simulink subsystem "Final_Project_PreRealSurface_20260605_142446"  (R2024a)
settings: Solver=VariableStepAuto  StartTime=0.0  StopTime=10.0  RelTol=1e-3
values from neighbouring files (symbols this model uses):
  D = hypot(Ep(:,1)-Tp(:,1)',Ep(:,2)-Tp(:,2)')    [pp_compare_stage.m]    (also in pp_diag_path.m; pp_t09_clear.m = hypot(Ep(:,1)-Tperim(:,1)', Ep(:,2)-Tperim(:,2)'); pp_tune2.m)
undefined symbols (not defined in the file or in its folder): waypoint_const
libraries: CarMaker4SL x83, simulink x2
(part 1 of 5)
settings Model: Creator=junho.lee  LastModifiedBy=hajin

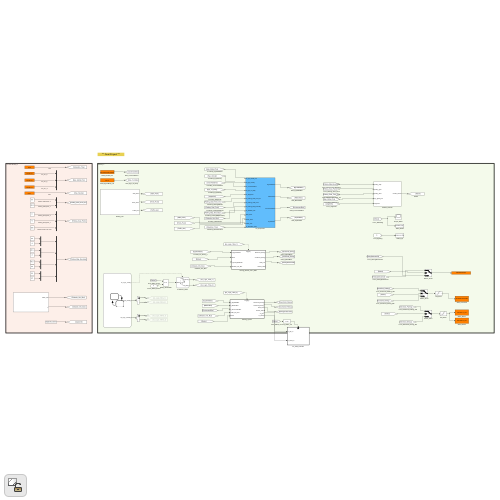
[thumbnail: Simulink's stored preview of the top-level diagram]
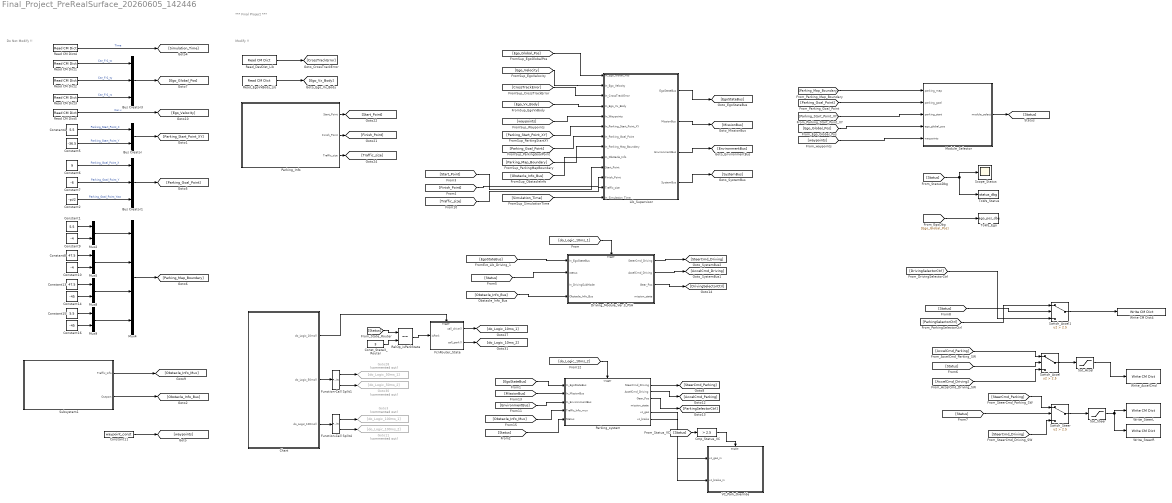
== system Final_Project_PreRealSurface_20260605_142446 ==
  note: Do Not Modify !!
  note: *** Final Project ***
  note: Modify !!
  Bus Creator : BusCreator  Inputs=2
  Bus Creator1 : BusCreator  Inputs=3
  Bus Creator3 : BusCreator  Inputs=3
  Chart : Stateflow chart  TreatAsAtomicUnit=on
  Cmp_Status_VC : simulink/Logic and Bit Operations/Compare To Constant  relop=>  const=2.5  OutDataTypeStr=boolean
  Const_State3_Router : Constant  Value=3
  Constant1 : Constant  Value=5.5
  Constant10 : Constant  Value=-4
  Constant11 : Constant  Value=waypoint_const
  Constant13 : Constant  Value=47.5
  Constant14 : Constant  Value=-45
  Constant15 : Constant  Value=5.5
  Constant16 : Constant  Value=-45
  Constant2 : Constant  Value=-pi/2
  Constant4 : Constant  Value=5.5
  Constant5 : Constant  Value=-36.5
  Constant6 : Constant  Value=9
  Constant7 : Constant  Value=-6
  Constant8 : Constant  Value=47.5
  Constant9 : Constant  Value=-4
  Driving_Module_Ver.3_PSH : Subsystem
  FcnRouter_State : Stateflow chart  TreatAsAtomicUnit=on
  Function-Call Split1 : FunctionCallSplit  IconShape=distinctive  NumOutputPorts=2  OutputPortLayout=default
  Function-Call Split4 : FunctionCallSplit  IconShape=distinctive  NumOutputPorts=2  OutputPortLayout=default
  Goto11 : Goto  Commented=on  GotoTag=do_Logic_100ms_2
  Goto28 : Goto  Commented=on  GotoTag=do_Logic_50ms_1
  Goto3 : Goto  Commented=on  GotoTag=do_Logic_100ms_1
  Goto30 : Goto  Commented=on  GotoTag=do_Logic_50ms_2
  Lib_Supervisor : Subsystem
  Module_Selector : Subsystem
  Mux{2,5,8..9} (4 alike) : Mux  Inputs=2
  Mux4 : Mux
  Parking_Info : Subsystem
  Parking_system : Subsystem
  Read CM Dict1 : CarMaker4SL/Read CM Dict  xname=Car.Fr1.tx  xsync=off  xstime=Inherited
  Read CM Dict2 : CarMaker4SL/Read CM Dict  xname=Car.Fr1.ty  xsync=off  xstime=Inherited
  Read CM Dict3 : CarMaker4SL/Read CM Dict  xname=Car.Fr1.rz  xsync=off  xstime=Inherited
  Read CM Dict4 : CarMaker4SL/Read CM Dict  xname=Time  xsync=off  xstime=Inherited
  Read CM Dict5 : CarMaker4SL/Read CM Dict  xname=Car.v  xsync=off  xstime=Inherited
  Read_DevDist_Lib : CarMaker4SL/Read CM Dict  xname=Car.Road.Path.DevDist  xsync=off  xstime=Inherited
  Read_EgoVxBody_Lib : CarMaker4SL/Read CM Dict  xname=Car.vx  xsync=off  xstime=Inherited
  RelOp_isParkState : RelationalOperator  Operator===
  Sat_Accel : Saturate  UpperLimit=3.0  LowerLimit=-5.0
  Sat_Steer : Saturate  UpperLimit=pi/6  LowerLimit=-pi/6
  Scope_Status : Scope
  Subsystem1 : Subsystem
  Switch_Accel : Switch  Criteria=u2 > Threshold  Threshold=2.5
  Switch_Accel1 : Switch  Criteria=u2 > Threshold  Threshold=2.5
  Switch_Steer : Switch  Criteria=u2 > Threshold  Threshold=2.5
  ToWs_Ego : ToWorkspace  VariableName=ego_pos_dbg  SaveFormat=Timeseries  SampleTime=-1
  ToWs_Status : ToWorkspace  VariableName=status_dbg  SaveFormat=Timeseries  SampleTime=-1
  VC_Park_Override : Subsystem
  Write CM Dict4 : CarMaker4SL/Write CM Dict  xname=DM.SelectorCtrl  xsync=off
  Write_AccelCmd : CarMaker4SL/Write CM Dict  xname=AccelCtrl.DesiredAx  xsync=off
  Write_SteerL : CarMaker4SL/Write CM Dict  xname=Car.CFL.rz_ext  xsync=off
  Write_SteerR : CarMaker4SL/Write CM Dict  xname=Car.CFR.rz_ext  xsync=off
  wires:
  Constant13/1 -> Mux8/1
  Subsystem1/1(Traffic_Info) -> [Obstacle_Info_Mux]
  Read CM Dict1/1 -> Bus Creator3/1  "Car_Fr1_tx"
  Read CM Dict3/1 -> Bus Creator3/3  "Car_Fr1_rz"
  Constant4/1 -> Bus Creator/1  "Parking_Start_Point_X"
  Chart/2(do_Logic_50ms()) -> Function-Call Split1/1
  Function-Call Split1/2 -> Goto30/1
  Read CM Dict4/1 -> [Simulation_Time]  "Time"
  Constant9/1 -> Mux2/2
  Bus Creator1/1 -> [Parking_Goal_Point]
  Mux8/1 -> Mux4/3
  Constant6/1 -> Bus Creator1/1  "Parking_Goal_Point_X"
  Constant1/1 -> Mux2/1
  Constant16/1 -> Mux9/2
  Read CM Dict2/1 -> Bus Creator3/2  "Car_Fr1_ty"
  Function-Call Split1/1 -> Goto28/1
  Constant5/1 -> Bus Creator/2  "Parking_Start_Point_Y"
  Constant7/1 -> Bus Creator1/2  "Parking_Goal_Point_Y"
  Read CM Dict5/1 -> [Ego_Velocity]  "Car.v"
  Constant15/1 -> Mux9/1
  Constant10/1 -> Mux5/2
  Bus Creator3/1 -> [Ego_Global_Pos]
  Constant14/1 -> Mux8/2
  Bus Creator/1 -> [Parking_Start_Point_XY]
  Mux9/1 -> Mux4/4
  Mux2/1 -> Mux4/1
  Mux4/1 -> [Parking_Map_Boundary]
  Constant8/1 -> Mux5/1
  Constant2/1 -> Bus Creator1/3  "Parking_Goal_Point_Yaw"
  Mux5/1 -> Mux4/2
  Chart/3(do_Logic_100ms()) -> Function-Call Split4/1
  Function-Call Split4/1 -> Goto3/1
  Function-Call Split4/2 -> Goto11/1
  Sat_Steer/1 -> Write_SteerR/1, Write_SteerL/1
  Read_DevDist_Lib/1 -> [CrossTrackError]
  Read_EgoVxBody_Lib/1 -> [Ego_Vx_Body]
  [Ego_Global_Pos] -> Lib_Supervisor/1(In_Ego_Global_Pos)
  [Ego_Velocity] -> Lib_Supervisor/2(In_Ego_Velocity)
  [CrossTrackError] -> Lib_Supervisor/3(In_CrossTrackError)
  [Ego_Vx_Body] -> Lib_Supervisor/4(In_Ego_Vx_Body)
  [waypoints] -> Lib_Supervisor/5(In_Waypoints)
  [Parking_Start_Point_XY] -> Lib_Supervisor/6(In_Parking_Start_Point_XY)
  [Parking_Goal_Point] -> Lib_Supervisor/7(In_Parking_Goal_Point)
  [Parking_Map_Boundary] -> Lib_Supervisor/8(In_Parking_Map_Boundary)
  [Simulation_Time] -> Lib_Supervisor/13(In_Simulation_Time)
  Lib_Supervisor/1(EgoStateBus) -> [EgoStateBus]
  Lib_Supervisor/2(MissionBus) -> [MissionBus]
  Lib_Supervisor/3(EnvironmentBus) -> [EnvironmentBus]
  Lib_Supervisor/4(SystemBus) -> [SystemBus]
  [EgoStateBus] -> Driving_Module_Ver.3_PSH/1(In_EgoStateBus)
  [do_Logic_10ms_1] -> Driving_Module_Ver.3_PSH/Trigger
  [SteerCmd_Parking] -> Switch_Steer/1
  [Status] -> Switch_Steer/2
  [SteerCmd_Driving] -> Switch_Steer/3
  Switch_Steer/1 -> Sat_Steer/1
  [AccelCmd_Parking] -> Switch_Accel/1
  [Status] -> Switch_Accel/2
  [AccelCmd_Driving] -> Switch_Accel/3
  Switch_Accel/1 -> Sat_Accel/1
  Switch_Accel1/1 -> Write CM Dict4/1
  Sat_Accel/1 -> Write_AccelCmd/1
  Subsystem1/2(Outport) -> [Obstacle_Info_Bus]
  [Obstacle_Info_Bus] -> Lib_Supervisor/9(In_Obstacle_Info)
  Driving_Module_Ver.3_PSH/1(SteerCmd_Driving) -> [SteerCmd_Driving]
  Driving_Module_Ver.3_PSH/2(AccelCmd_Driving) -> [AccelCmd_Driving]
  [Obstacle_Info_Bus] -> Driving_Module_Ver.3_PSH/4(Obstacle_Info_Bus)
  Driving_Module_Ver.3_PSH/3(Gear_Pos) -> [DrivingSelectorCtrl]
  Parking_Info/1(Start_Point) -> [Start_Point]
  Parking_Info/2(Finish_Point) -> [Finish_Point]
  Parking_Info/3(Traffic_size) -> [Traffic_size]
  [Start_Point] -> Lib_Supervisor/10(Start_Point)
  [Finish_Point] -> Lib_Supervisor/11(Finish_Point)
  [Traffic_size] -> Lib_Supervisor/12(Traffic_size)
  [do_Logic_10ms_2] -> Parking_system/Trigger
  [EgoStateBus] -> Parking_system/1(In_EgoStateBus)
  [EnvironmentBus] -> Parking_system/3(In_EnvironmentBus)
  [MissionBus] -> Parking_system/2(In_MissionBus)
  [Obstacle_Info_Mux] -> Parking_system/4(Traffic_Info_mux)
  [Status] -> Driving_Module_Ver.3_PSH/2(status)
  [Parking_Map_Boundary] -> Module_Selector/1(parking_map)
  [Parking_Goal_Point] -> Module_Selector/2(parking_goal)
  [Parking_Start_Point_XY] -> Module_Selector/3(parking_start)
  [Ego_Global_Pos] -> Module_Selector/4(ego_global_pos)
  [waypoints] -> Module_Selector/5(waypoints)
  Module_Selector/1(module_select) -> [Status]
  [Status] -> Parking_system/5(Status)
  Constant11/1 -> [waypoints]
  [Status] -> Scope_Status/1, ToWs_Status/1
  [Ego_Global_Pos] -> ToWs_Ego/1
  [Status] -> RelOp_isParkState/1
  Const_State3_Router/1 -> RelOp_isParkState/2
  Chart/1(do_Logic_10ms()) -> FcnRouter_State/Trigger
  RelOp_isParkState/1 -> FcnRouter_State/1(isPark)
  FcnRouter_State/1(call_drive()) -> [do_Logic_10ms_1]
  FcnRouter_State/2(call_park()) -> [do_Logic_10ms_2]
  [Status] -> Switch_Accel1/2
  Parking_system/1(SteerCmd_Driving) -> [SteerCmd_Parking]
  Parking_system/2(AccelCmd_Driving) -> [AccelCmd_Parking]
  Parking_system/3(Gear_Pos) -> [ParkingSelectorCtrl]
  [ParkingSelectorCtrl] -> Switch_Accel1/1
  [DrivingSelectorCtrl] -> Switch_Accel1/3
  [Status] -> Cmp_Status_VC/1
  Cmp_Status_VC/1 -> VC_Park_Override/Enable
  Parking_system/5(vc_gas) -> VC_Park_Override/1(vc_gas_in)
  Parking_system/6(vc_brake) -> VC_Park_Override/2(vc_brake_in)

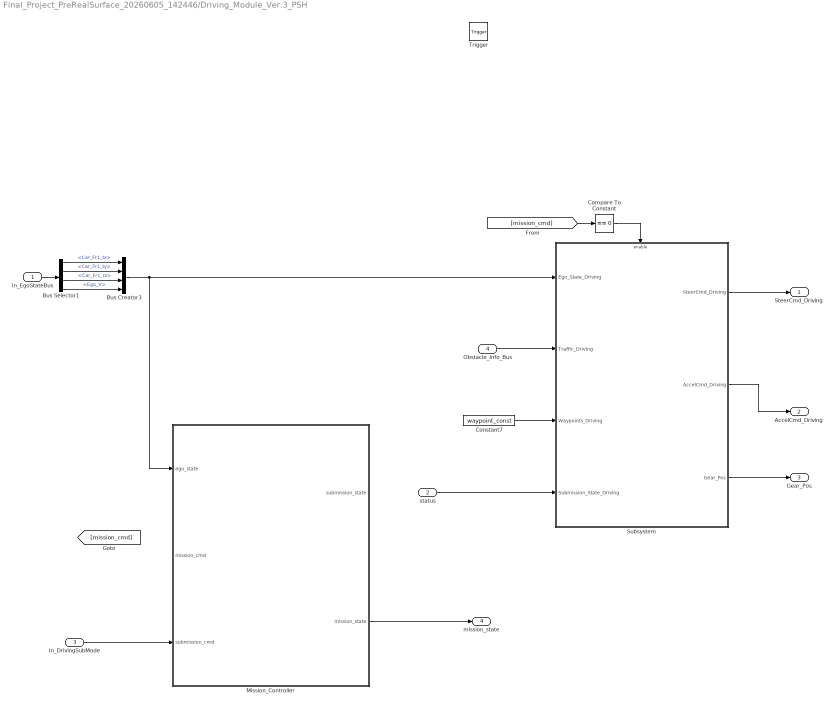
== system Final_Project_PreRealSurface_20260605_142446/Driving_Module_Ver.3_PSH ==
  In_EgoStateBus : Inport
  status : Inport  Port=2
  In_DrivingSubMode : Inport  Port=3
  Obstacle_Info_Bus : Inport  Port=4
  Trigger : TriggerPort  TriggerType=function-call  VariantControl=(inherit)
  Bus Creator3 : BusCreator  Inputs=4  OutDataTypeStr=Bus: EgoStateBus
  Bus Selector1 : BusSelector  OutputSignals=Car_Fr1_tx,Car_Fr1_ty,Car_Fr1_rz,Ego_V
  Compare To Constant : simulink/Logic and Bit Operations/Compare To Constant  relop===  const=0  OutDataTypeStr=boolean
  Constant7 : Constant  Value=waypoint_const
  Mission_Controller : MATLAB Function  TreatAsAtomicUnit=on
  Subsystem : Subsystem
  SteerCmd_Driving : Outport
  AccelCmd_Driving : Outport  Port=2
  Gear_Pos : Outport  Port=3
  mission_state : Outport  Port=4
  wires:
  status/1 -> Subsystem/4(Submission_State_Driving)
  Subsystem/3(Gear_Pos) -> Gear_Pos/1
  Compare To Constant/1 -> Subsystem/Enable
  [mission_cmd] -> Compare To Constant/1
  In_DrivingSubMode/1 -> Mission_Controller/3(submission_cmd)
  Mission_Controller/2(mission_state) -> mission_state/1
  In_EgoStateBus/1 -> Bus Selector1/1
  Bus Selector1/4 -> Bus Creator3/4  "<Ego_V>"
  Bus Creator3/1 -> Mission_Controller/1(ego_state), Subsystem/1(Ego_State_Driving)
  Bus Selector1/3 -> Bus Creator3/3  "<Car_Fr1_rz>"
  Bus Selector1/2 -> Bus Creator3/2  "<Car_Fr1_ty>"
  Bus Selector1/1 -> Bus Creator3/1  "<Car_Fr1_tx>"
  Constant7/1 -> Subsystem/3(Waypoints_Driving)
  Obstacle_Info_Bus/1 -> Subsystem/2(Traffic_Driving)
  Subsystem/2(AccelCmd_Driving) -> AccelCmd_Driving/1
  Subsystem/1(SteerCmd_Driving) -> SteerCmd_Driving/1

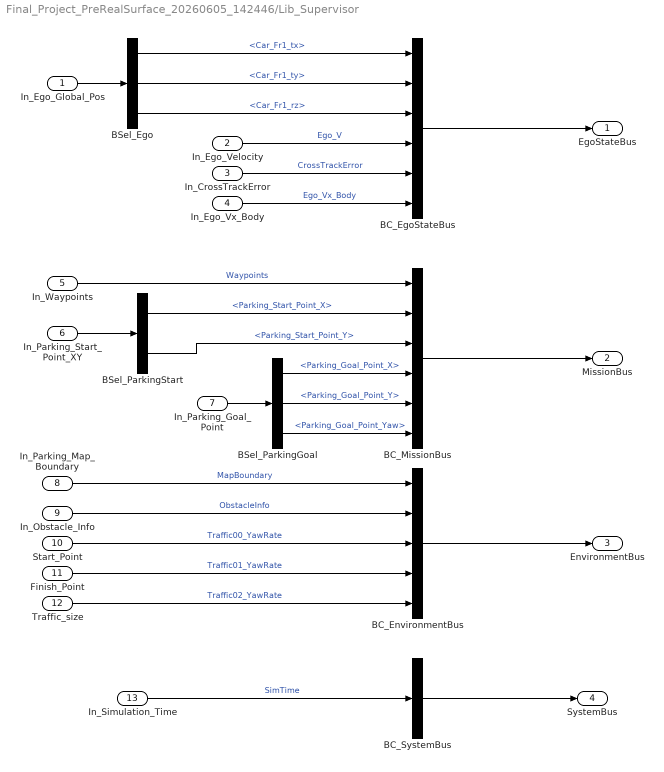
== system Final_Project_PreRealSurface_20260605_142446/Lib_Supervisor ==
  In_Ego_Global_Pos : Inport
  In_Ego_Velocity : Inport  Port=2
  In_CrossTrackError : Inport  Port=3
  In_Ego_Vx_Body : Inport  Port=4
  In_Waypoints : Inport  Port=5
  In_Parking_Start_Point_XY : Inport  Port=6
  In_Parking_Goal_Point : Inport  Port=7
  In_Parking_Map_Boundary : Inport  Port=8
  In_Obstacle_Info : Inport  Port=9
  Start_Point : Inport  Port=10
  Finish_Point : Inport  Port=11
  Traffic_size : Inport  Port=12
  In_Simulation_Time : Inport  Port=13
  BC_EgoStateBus : BusCreator  Inputs=6
  BC_EnvironmentBus : BusCreator  Inputs=5
  BC_MissionBus : BusCreator  Inputs=6
  BC_SystemBus : BusCreator  Inputs=1
  BSel_Ego : BusSelector  OutputSignals=Car_Fr1_tx,Car_Fr1_ty,Car_Fr1_rz
  BSel_ParkingGoal : BusSelector  OutputSignals=Parking_Goal_Point_X,Parking_Goal_Point_Y,Parking_Goal_Point_Yaw
  BSel_ParkingStart : BusSelector  OutputSignals=Parking_Start_Point_X,Parking_Start_Point_Y
  EgoStateBus : Outport
  MissionBus : Outport  Port=2
  EnvironmentBus : Outport  Port=3
  SystemBus : Outport  Port=4
  wires:
  In_Ego_Global_Pos/1 -> BSel_Ego/1
  In_Parking_Start_Point_XY/1 -> BSel_ParkingStart/1
  In_Parking_Goal_Point/1 -> BSel_ParkingGoal/1
  BSel_Ego/1 -> BC_EgoStateBus/1  "<Car_Fr1_tx>"
  BSel_Ego/2 -> BC_EgoStateBus/2  "<Car_Fr1_ty>"
  BSel_Ego/3 -> BC_EgoStateBus/3  "<Car_Fr1_rz>"
  In_Ego_Velocity/1 -> BC_EgoStateBus/4  "Ego_V"
  In_CrossTrackError/1 -> BC_EgoStateBus/5  "CrossTrackError"
  In_Ego_Vx_Body/1 -> BC_EgoStateBus/6  "Ego_Vx_Body"
  In_Waypoints/1 -> BC_MissionBus/1  "Waypoints"
  BSel_ParkingStart/1 -> BC_MissionBus/2  "<Parking_Start_Point_X>"
  BSel_ParkingStart/2 -> BC_MissionBus/3  "<Parking_Start_Point_Y>"
  BSel_ParkingGoal/1 -> BC_MissionBus/4  "<Parking_Goal_Point_X>"
  BSel_ParkingGoal/2 -> BC_MissionBus/5  "<Parking_Goal_Point_Y>"
  BSel_ParkingGoal/3 -> BC_MissionBus/6  "<Parking_Goal_Point_Yaw>"
  In_Parking_Map_Boundary/1 -> BC_EnvironmentBus/1  "MapBoundary"
  In_Obstacle_Info/1 -> BC_EnvironmentBus/2  "ObstacleInfo"
  Start_Point/1 -> BC_EnvironmentBus/3  "Traffic00_YawRate"
  Finish_Point/1 -> BC_EnvironmentBus/4  "Traffic01_YawRate"
  Traffic_size/1 -> BC_EnvironmentBus/5  "Traffic02_YawRate"
  In_Simulation_Time/1 -> BC_SystemBus/1  "SimTime"
  BC_EgoStateBus/1 -> EgoStateBus/1
  BC_MissionBus/1 -> MissionBus/1
  BC_EnvironmentBus/1 -> EnvironmentBus/1
  BC_SystemBus/1 -> SystemBus/1

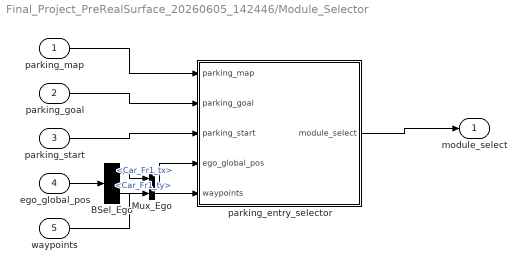
== system Final_Project_PreRealSurface_20260605_142446/Module_Selector ==
  parking_map : Inport
  parking_goal : Inport  Port=2
  parking_start : Inport  Port=3
  ego_global_pos : Inport  Port=4
  waypoints : Inport  Port=5
  BSel_Ego : BusSelector  OutputSignals=Car_Fr1_tx,Car_Fr1_ty
  Mux_Ego : Mux  Inputs=2
  parking_entry_selector : MATLAB Function  TreatAsAtomicUnit=on
  module_select : Outport
  wires:
  parking_map/1 -> parking_entry_selector/1(parking_map)
  parking_goal/1 -> parking_entry_selector/2(parking_goal)
  parking_start/1 -> parking_entry_selector/3(parking_start)
  waypoints/1 -> parking_entry_selector/5(waypoints)
  parking_entry_selector/1(module_select) -> module_select/1
  ego_global_pos/1 -> BSel_Ego/1
  BSel_Ego/1 -> Mux_Ego/1  "<Car_Fr1_tx>"
  BSel_Ego/2 -> Mux_Ego/2  "<Car_Fr1_ty>"
  Mux_Ego/1 -> parking_entry_selector/4(ego_global_pos)

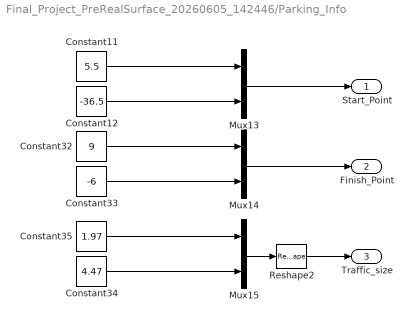
== system Final_Project_PreRealSurface_20260605_142446/Parking_Info ==
  Constant11 : Constant  Value=5.5
  Constant12 : Constant  Value=-36.5
  Constant32 : Constant  Value=9
  Constant33 : Constant  Value=-6
  Constant34 : Constant  Value=4.47
  Constant35 : Constant  Value=1.97
  Mux13 : Mux  Inputs=2
  Mux14 : Mux  Inputs=2
  Mux15 : Mux  Inputs=2
  Reshape2 : Reshape  OutputDimensionality=Row vector (2-D)  OutputDimensions=[2,2]
  Start_Point : Outport
  Finish_Point : Outport  Port=2
  Traffic_size : Outport  Port=3
  wires:
  Constant12/1 -> Mux13/2
  Constant11/1 -> Mux13/1
  Constant33/1 -> Mux14/2
  Mux13/1 -> Start_Point/1
  Reshape2/1 -> Traffic_size/1
  Mux15/1 -> Reshape2/1
  Constant32/1 -> Mux14/1
  Constant34/1 -> Mux15/2
  Constant35/1 -> Mux15/1
  Mux14/1 -> Finish_Point/1

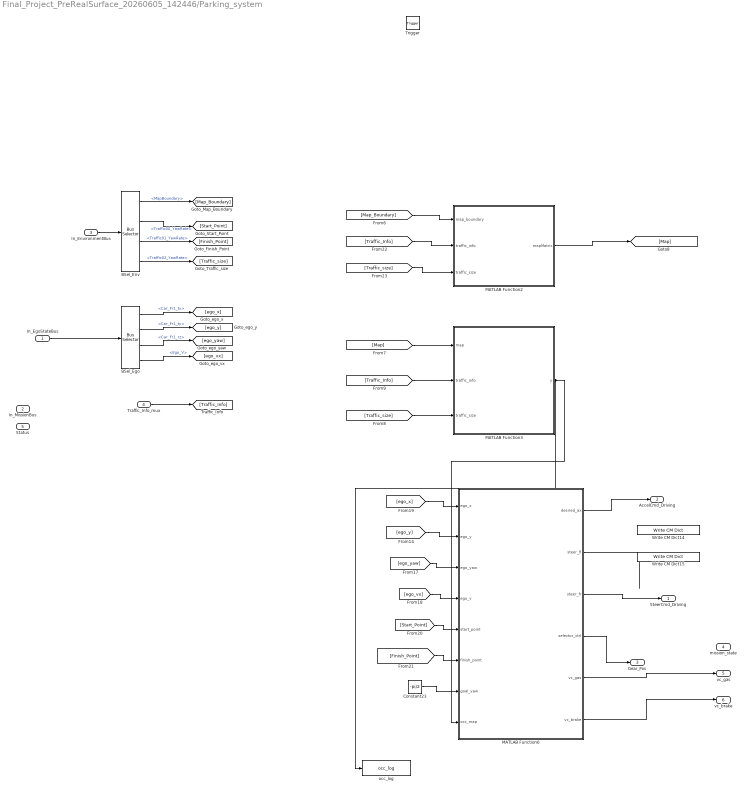
== system Final_Project_PreRealSurface_20260605_142446/Parking_system ==
  In_EgoStateBus : Inport
  In_MissionBus : Inport  Port=2
  In_EnvironmentBus : Inport  Port=3
  Traffic_Info_mux : Inport  Port=4
  Status : Inport  Port=5
  Trigger : TriggerPort  TriggerType=function-call  VariantControl=(inherit)
  BSel_Ego : BusSelector  OutputSignals=Car_Fr1_tx,Car_Fr1_ty,Car_Fr1_rz,Ego_V
  BSel_Env : BusSelector  OutputSignals=MapBoundary,Traffic00_YawRate,Traffic01_YawRate,Traffic02_YawRate
  Constant23 : Constant  Value=-pi/2
  MATLAB Function2 : MATLAB Function  TreatAsAtomicUnit=on
  MATLAB Function3 : MATLAB Function  TreatAsAtomicUnit=on
  MATLAB Function6 : MATLAB Function  TreatAsAtomicUnit=on
  Write CM Dict14 : CarMaker4SL/Write CM Dict  xname=Car.CFL.rz_ext  xsync=off
  Write CM Dict15 : CarMaker4SL/Write CM Dict  xname=Car.CFR.rz_ext  xsync=off
  occ_log : ToWorkspace  VariableName=occ_log  SaveFormat=Timeseries  SampleTime=-1
      settings: MaxDataPoints=1  Decimation=3000
  SteerCmd_Driving : Outport
  AccelCmd_Driving : Outport  Port=2
  Gear_Pos : Outport  Port=3
  mission_state : Outport  Port=4
  vc_gas : Outport  Port=5
  vc_brake : Outport  Port=6
  wires:
  [Finish_Point] -> MATLAB Function6/6(finish_point)
  Constant23/1 -> MATLAB Function6/7(goal_yaw)
  MATLAB Function6/4(selector_ctrl) -> Gear_Pos/1
  MATLAB Function6/3(steer_fr) -> SteerCmd_Driving/1
  MATLAB Function6/2(steer_fl) -> ?
  MATLAB Function3/1(y) -> MATLAB Function6/8(occ_map), occ_log/1
  Traffic_Info_mux/1 -> [Traffic_Info]
  MATLAB Function6/1(desired_ax) -> AccelCmd_Driving/1
  [Start_Point] -> MATLAB Function6/5(start_point)
  [ego_vx] -> MATLAB Function6/4(ego_v)
  [ego_yaw] -> MATLAB Function6/3(ego_yaw)
  [ego_y] -> MATLAB Function6/2(ego_y)
  [ego_x] -> MATLAB Function6/1(ego_x)
  [Traffic_size] -> MATLAB Function3/3(traffic_size)
  [Traffic_Info] -> MATLAB Function3/2(traffic_info)
  [Map] -> MATLAB Function3/1(map)
  MATLAB Function2/1(mapMatrix) -> [Map]
  [Traffic_size] -> MATLAB Function2/3(traffic_size)
  [Traffic_Info] -> MATLAB Function2/2(traffic_info)
  [Map_Boundary] -> MATLAB Function2/1(map_boundary)
  In_EgoStateBus/1 -> BSel_Ego/1
  In_EnvironmentBus/1 -> BSel_Env/1
  BSel_Ego/1 -> [ego_x]  "<Car_Fr1_tx>"
  BSel_Ego/2 -> [ego_y]  "<Car_Fr1_ty>"
  BSel_Ego/3 -> [ego_yaw]  "<Car_Fr1_rz>"
  BSel_Ego/4 -> [ego_vx]  "<Ego_V>"
  BSel_Env/1 -> [Map_Boundary]  "<MapBoundary>"
  BSel_Env/2 -> [Start_Point]  "<Traffic00_YawRate>"
  BSel_Env/3 -> [Finish_Point]  "<Traffic01_YawRate>"
  BSel_Env/4 -> [Traffic_size]  "<Traffic02_YawRate>"
  MATLAB Function6/5(vc_gas) -> vc_gas/1
  MATLAB Function6/6(vc_brake) -> vc_brake/1
